simulink model "diff"  (R2023a)
settings: Solver=VariableStepAuto  StartTime=0.0  StopTime=10.0  RelTol=1e-3
libraries: slpidlib x3, embmathops x2
settings Model: Creator=Ahmed  LastModifiedBy=Ahmed

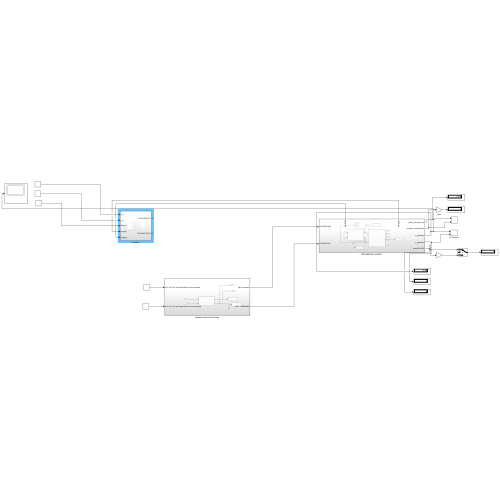
[thumbnail: Simulink's stored preview of the top-level diagram]
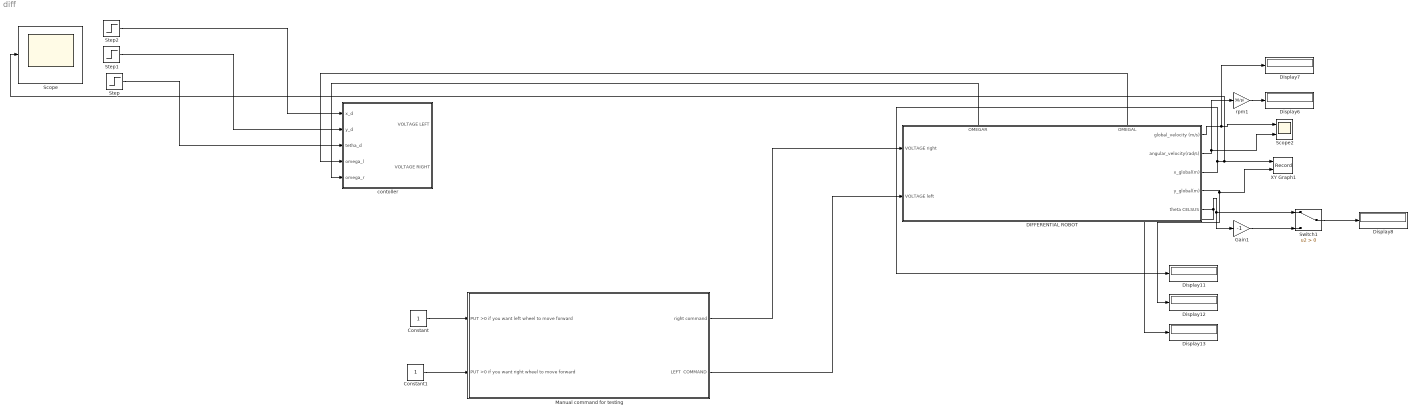
== system diff ==
  Constant : Constant
  Constant1 : Constant
  "DIFFERENTIAL ROBOT " : Subsystem
      settings: PortSchema="{\"entries\":[{\"content\":{\"sides\":[{\"content\":{\"connectorIds\":[\"In1\",\"In2\"]},\"type\":\"ConnectorPlacement.EquallySpacedRectSide\",\"uuid\":\"391234ff-cfec-4f6c-a138-89dd313d7130\"},{\"content\":{\"connectorIds\":[\"Out1\",\"Out2\",\"Out3\",\"Out4\",\"Out5\"],\"side\":\"RIGHT\"},\"type\":\"ConnectorPlacement.EquallySpacedRectSide\",\"uuid\":\"b1b937cc-f74e-4d9f-a8b8-80c8e8e7239a\"},{\"content\":{\"connectorIds\":[\"Out6\",\"Out7\"],\"side\":\"TOP\"},\"type\":\"ConnectorPlacement.EquallySpacedRectSide\",\"uuid\":\"bef0db1f-016c-4d9f-9b1d-66f8cf7cef5e\"}]},\"type\":\"ConnectorPlacement.EquallySpacedConnector\",\"uuid\":\"3118eaf9-68a7-431f-bc06-97b9db44cc22\"}],\"packageUris\":[\"http://schema.mathworks.com/mf0/Connector/R2020b\"],\"version\":\"1.0\"}"
  Display{6..8,11..13} (6 alike) : Display
  Gain1 : Gain  Gain=-1
  Manual command for testing : Subsystem
  Scope : Scope
  Scope2 : Scope  NumInputPorts=2
  Step : Step  After=0  SampleTime=0
  Step1 : Step  SampleTime=0
  Step2 : Step  SampleTime=0
  Switch1 : Switch  Criteria=u2 > Threshold  SaturateOnIntegerOverflow=off  InputSameDT=off
  XY Graph1 : Record  FileSettingsInternal="{\"entries\":[{\"content\":{\"excelSettings\":{\"content\":{},\"type\":\"Streamout.ExcelSettings\"}},\"type\":\"Streamout.FileSettingStorage\",\"uuid\":\"2b7d8dd8-c0b9-49d7-b7ba-ae24f0353f97\"}],\"packageUris\":[\"http://schema.mathworks.com/mf0/streamout_blocks/R2020a\"],\"version\":\"1.0\"}"  Layout=[1 1]  SignalsInternal="{\"entries\":[{\"content\":{\"signals\":[{\"content\":{\"blockPath\":[\"diff/XY Graph1\"],\"dimensions\":[1],\"domain\":\"diff/XY Graph1\",\"lineColor\":\"#a2142f\",\"plots\":[1],\"port\":1,\"sid\":[\"\"],\"signalID\":19857,\"signalName\":\"DIFERENTIAL ROBOT SYSTEM1:3\"},\"type\":\"RecordBlkView.Signal\",\"uuid\":\"70d8382d-8876-4a89-8d0a-8a042afd1f92\"},{\"content\":{\"blockPath\":[\"diff/XY Graph1\"],\"dimensions\":[1],\"domain\":\"diff/XY Graph1\",\"lineColor\":\"#139fff\",\"plots\":[1],\"port\":2,\"sid\":[\"\"],\"signalID\":19861,\"signalName\":\"DIFERENTIAL ROBOT SYSTEM1:4\"},\"type\":\"RecordBlkView.Signal\",\"uuid\":\"2fa1e0bd-1433-42a0-a5d9-6edbe41dc125\"}]},\"type\":\"RecordBlkView.InputSignals\",\"uuid\":\"f1bdc88a-c7a9-4fa2-8817-dae53eaa0189\"}],\"packageUris\":[\"http://schema.mathworks.com/mf0/streamout_blocks/R2020a\"],\"version\":\"1.0\"}"  VisualizationBindings="{\"xyplotplugin\":{\"info\":[{\"series\":[{\"bindingParametersList\":[{\"parameter\":\"X-Axis\",\"signalID\":19857,\"signalName\":\"DIFERENTIAL ROBOT SYSTEM1:3\"},{\"parameter\":\"Y-Axis\",\"signalID\":19861,\"signalName\":\"DIFERENTIAL ROBOT SYSTEM1:4\"}],\"seriesID\":42501}],\"subplotID\":1}]}}"  CompatibilityTag=XY
  contoller : Subsystem
  rpm1 : Gain  Gain=30/pi
  wires:
  Manual command for testing/1(right command) -> "DIFFERENTIAL ROBOT "/1(VOLTAGE right)
  Step2/1 -> contoller/1(x_d)
  Step1/1 -> contoller/2(y_d)
  Constant1/1 -> Manual command for testing/2(PUT >0 if you want right wheel to move forward)
  Step/1 -> contoller/3(tetha_d)
  "DIFFERENTIAL ROBOT "/6(OMEGAR) -> contoller/5(omega_r)
  Manual command for testing/2(LEFT  COMMAND) -> "DIFFERENTIAL ROBOT "/2(VOLTAGE left)
  "DIFFERENTIAL ROBOT "/2(angular_velocity(rad/s)) -> rpm1/1, Scope2/2
  "DIFFERENTIAL ROBOT "/1(global_velocity (m/s)) -> Display7/1, Scope2/1
  Switch1/1 -> Display8/1
  "DIFFERENTIAL ROBOT "/5(theta CELSUS) -> Gain1/1, Switch1/1, Display13/1
  Gain1/1 -> Switch1/3
  "DIFFERENTIAL ROBOT "/4(y_global(m)) -> XY Graph1/2, Display12/1
  "DIFFERENTIAL ROBOT "/7(OMEGAL) -> contoller/4(omega_l)
  rpm1/1 -> Display6/1
  "DIFFERENTIAL ROBOT "/3(x_global(m)) -> Display11/1, XY Graph1/1, Scope/1
  Constant/1 -> Manual command for testing/1(PUT >0 if you want left wheel to move forward)

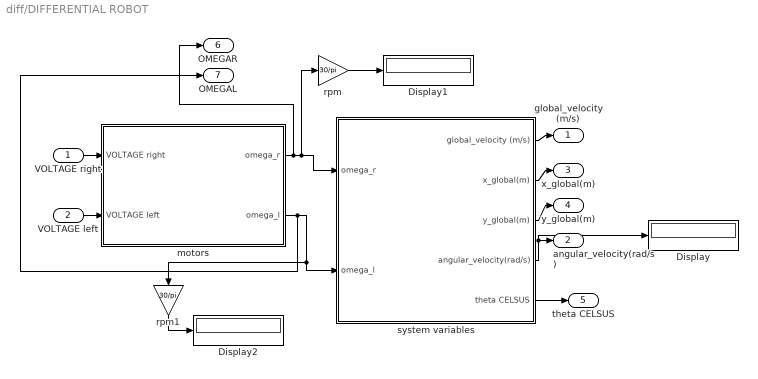
== system diff/DIFFERENTIAL ROBOT  ==
  VOLTAGE right : Inport
  VOLTAGE left : Inport  Port=2
  Display : Display
  Display1 : Display
  Display2 : Display
  motors : Subsystem
  rpm : Gain  Gain=30/pi
  rpm1 : Gain  Gain=30/pi
  system variables : Subsystem
  global_velocity (m/s) : Outport
  angular_velocity(rad/s) : Outport  Port=2
  x_global(m) : Outport  Port=3
  y_global(m) : Outport  Port=4
  theta CELSUS : Outport  Port=5
  OMEGAR : Outport  Port=6
  OMEGAL : Outport  Port=7
  wires:
  motors/1(omega_r) -> OMEGAR/1, rpm/1, system variables/1(omega_r)
  motors/2(omega_l) -> OMEGAL/1, rpm1/1, system variables/2(omega_l)
  system variables/1(global_velocity (m/s)) -> global_velocity (m/s)/1
  system variables/2(x_global(m)) -> x_global(m)/1
  system variables/3(y_global(m)) -> y_global(m)/1
  VOLTAGE right/1 -> motors/1(VOLTAGE right)
  VOLTAGE left/1 -> motors/2(VOLTAGE left)
  system variables/4(angular_velocity(rad/s)) -> Display/1, angular_velocity(rad/s)/1
  system variables/5(theta CELSUS) -> theta CELSUS/1
  rpm/1 -> Display1/1
  rpm1/1 -> Display2/1

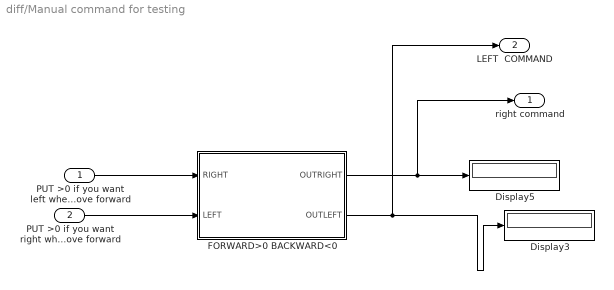
== system diff/Manual command for testing ==
  PUT >0 if you want left wheel to move forward : Inport
  PUT >0 if you want right wheel to move forward : Inport  Port=2
  Display3 : Display
  Display5 : Display
  FORWARD>0 BACKWARD<0 : Subsystem
  right command : Outport
  LEFT  COMMAND : Outport  Port=2
  wires:
  PUT >0 if you want left wheel to move forward/1 -> FORWARD>0 BACKWARD<0/1(RIGHT)
  FORWARD>0 BACKWARD<0/1(OUTRIGHT) -> right command/1, Display5/1
  FORWARD>0 BACKWARD<0/2(OUTLEFT) -> LEFT  COMMAND/1, Display3/1
  PUT >0 if you want right wheel to move forward/1 -> FORWARD>0 BACKWARD<0/2(LEFT)

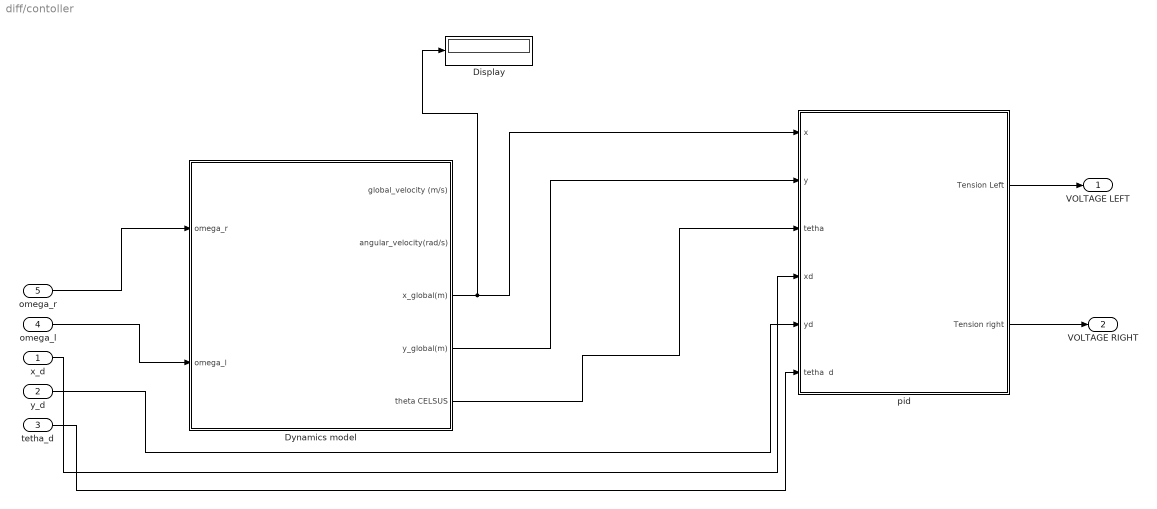
== system diff/contoller ==
  x_d : Inport
  y_d : Inport  Port=2
  tetha_d : Inport  Port=3
  omega_l : Inport  Port=4
  omega_r : Inport  Port=5
  Display : Display
  Dynamics model : Subsystem
  pid : Subsystem
  VOLTAGE LEFT : Outport
  VOLTAGE RIGHT : Outport  Port=2
  wires:
  Dynamics model/5(theta CELSUS) -> pid/3(tetha)
  Dynamics model/4(y_global(m)) -> pid/2(y)
  Dynamics model/3(x_global(m)) -> Display/1, pid/1(x)
  x_d/1 -> pid/4(xd)
  y_d/1 -> pid/5(yd)
  tetha_d/1 -> pid/6(tetha  d)
  omega_r/1 -> Dynamics model/1(omega_r)
  omega_l/1 -> Dynamics model/2(omega_l)
  pid/1(Tension Left) -> VOLTAGE LEFT/1
  pid/2(Tension right) -> VOLTAGE RIGHT/1

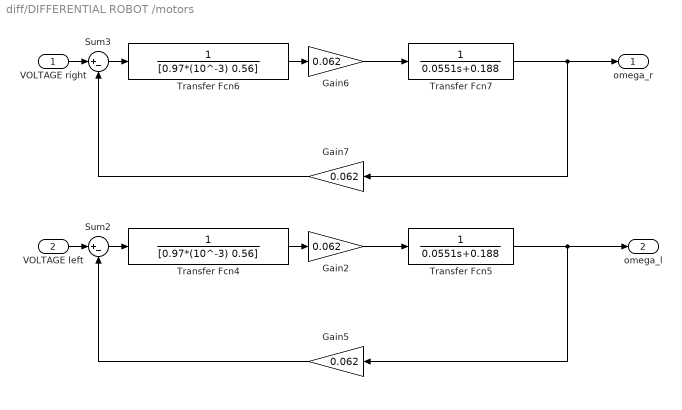
== system diff/DIFFERENTIAL ROBOT /motors ==
  VOLTAGE right : Inport
  VOLTAGE left : Inport  Port=2
  Gain{2,5..7} (4 alike) : Gain  Gain=0.062
  Sum2 : Sum  Inputs=|+-
  Sum3 : Sum  Inputs=|+-
  Transfer Fcn4 : TransferFcn  Denominator=[0.97*(10^-3) 0.56]
  Transfer Fcn5 : TransferFcn  Denominator=[0.0551 0.188]
  Transfer Fcn6 : TransferFcn  Denominator=[0.97*(10^-3) 0.56]
  Transfer Fcn7 : TransferFcn  Denominator=[0.0551 0.188]
  omega_r : Outport
  omega_l : Outport  Port=2
  wires:
  Transfer Fcn7/1 -> omega_r/1, Gain7/1
  Gain2/1 -> Transfer Fcn5/1
  Transfer Fcn5/1 -> omega_l/1, Gain5/1
  Gain6/1 -> Transfer Fcn7/1
  VOLTAGE left/1 -> Sum2/1
  Sum2/1 -> Transfer Fcn4/1
  Transfer Fcn6/1 -> Gain6/1
  Sum3/1 -> Transfer Fcn6/1
  Gain5/1 -> Sum2/2
  VOLTAGE right/1 -> Sum3/1
  Gain7/1 -> Sum3/2
  Transfer Fcn4/1 -> Gain2/1

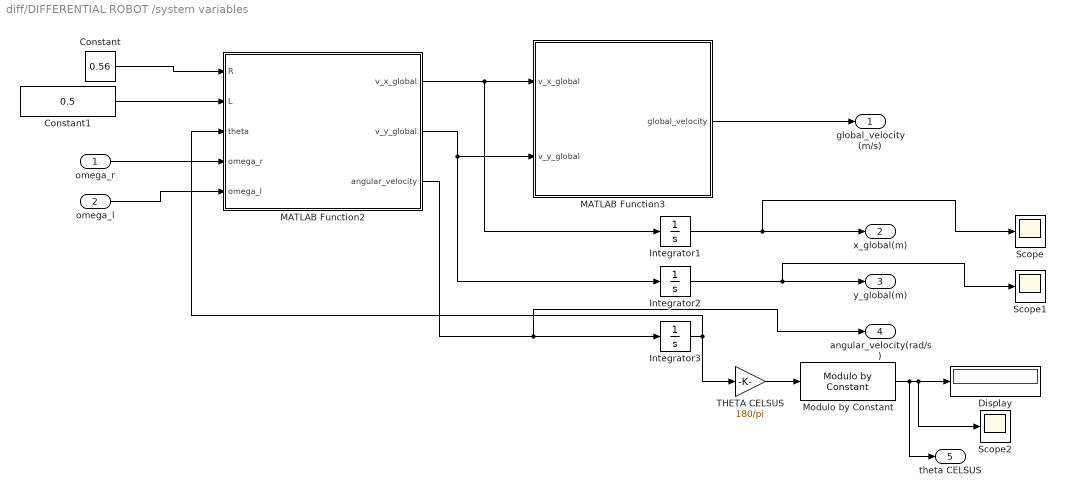
== system diff/DIFFERENTIAL ROBOT /system variables ==
  omega_r : Inport
  omega_l : Inport  Port=2
  Constant : Constant  Value=0.56
  Constant1 : Constant  Value=0.5
  Display : Display
  Integrator1 : Integrator
  Integrator2 : Integrator
  Integrator3 : Integrator
  MATLAB Function2 : MATLAB Function  TreatAsAtomicUnit=on
  MATLAB Function3 : MATLAB Function  TreatAsAtomicUnit=on
  Modulo by Constant : embmathops/Modulo by Constant  Denominator=360  SimulateUsing=Code generation
      settings: LibrarySourceBlock=embeddedMathLib/Modulo by Constant
  Scope : Scope
  Scope1 : Scope
  Scope2 : Scope
  THETA CELSUS : Gain  Gain=180/pi
  global_velocity (m/s) : Outport
  x_global(m) : Outport  Port=2
  y_global(m) : Outport  Port=3
  angular_velocity(rad/s) : Outport  Port=4
  theta CELSUS : Outport  Port=5
  wires:
  MATLAB Function2/3(angular_velocity) -> angular_velocity(rad/s)/1, Integrator3/1
  MATLAB Function2/1(v_x_global) -> Integrator1/1, MATLAB Function3/1(v_x_global)
  Constant1/1 -> MATLAB Function2/2(L)
  Integrator3/1 -> MATLAB Function2/3(theta), THETA CELSUS/1
  omega_l/1 -> MATLAB Function2/5(omega_l)
  MATLAB Function2/2(v_y_global) -> Integrator2/1, MATLAB Function3/2(v_y_global)
  Constant/1 -> MATLAB Function2/1(R)
  omega_r/1 -> MATLAB Function2/4(omega_r)
  Integrator2/1 -> Scope1/1, y_global(m)/1
  Integrator1/1 -> Scope/1, x_global(m)/1
  MATLAB Function3/1(global_velocity) -> global_velocity (m/s)/1
  Modulo by Constant/1 -> theta CELSUS/1, Display/1, Scope2/1
  THETA CELSUS/1 -> Modulo by Constant/1

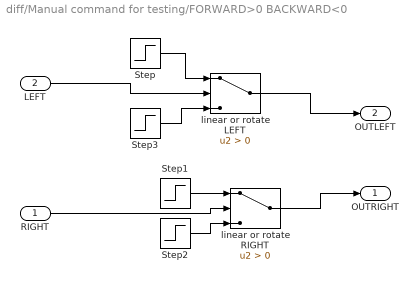
== system diff/Manual command for testing/FORWARD>0 BACKWARD<0 ==
  RIGHT : Inport
  LEFT : Inport  Port=2
  Step : Step  After=12  SampleTime=0
  Step1 : Step  After=12  SampleTime=0
  Step2 : Step  After=-12  SampleTime=0
  Step3 : Step  After=-12  SampleTime=0
  linear or rotate LEFT : Switch  Criteria=u2 > Threshold  SaturateOnIntegerOverflow=off  InputSameDT=off
  "linear or rotate RIGHT " : Switch  Criteria=u2 > Threshold  SaturateOnIntegerOverflow=off  InputSameDT=off
  OUTRIGHT : Outport
  OUTLEFT : Outport  Port=2
  wires:
  Step1/1 -> "linear or rotate RIGHT "/1
  "linear or rotate RIGHT "/1 -> OUTRIGHT/1
  Step2/1 -> "linear or rotate RIGHT "/3
  RIGHT/1 -> "linear or rotate RIGHT "/2
  Step3/1 -> linear or rotate LEFT/3
  Step/1 -> linear or rotate LEFT/1
  linear or rotate LEFT/1 -> OUTLEFT/1
  LEFT/1 -> linear or rotate LEFT/2

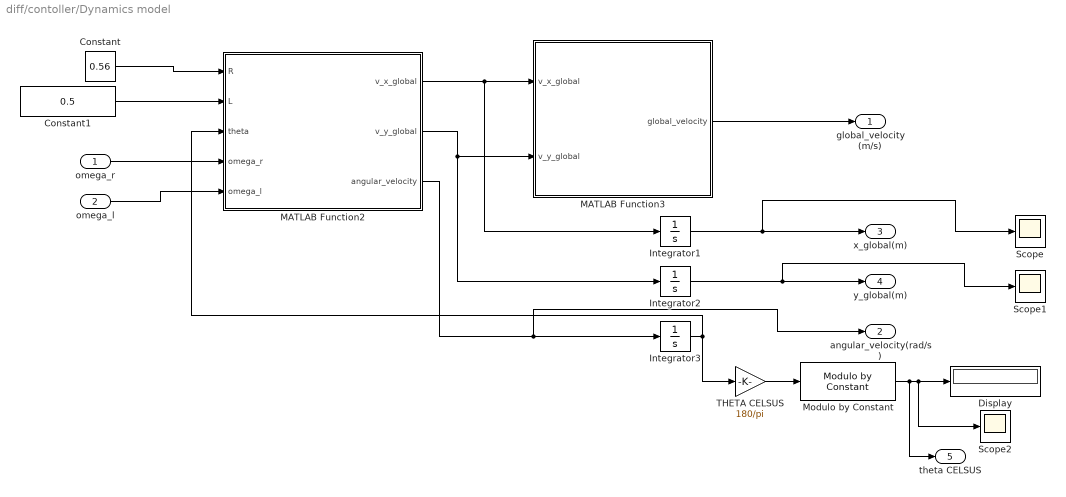
== system diff/contoller/Dynamics model ==
  omega_r : Inport
  omega_l : Inport  Port=2
  Constant : Constant  Value=0.56
  Constant1 : Constant  Value=0.5
  Display : Display
  Integrator1 : Integrator
  Integrator2 : Integrator
  Integrator3 : Integrator
  MATLAB Function2 : MATLAB Function  TreatAsAtomicUnit=on
  MATLAB Function3 : MATLAB Function  TreatAsAtomicUnit=on
  Modulo by Constant : embmathops/Modulo by Constant  Denominator=360  SimulateUsing=Code generation
      settings: LibrarySourceBlock=embeddedMathLib/Modulo by Constant
  Scope : Scope
  Scope1 : Scope
  Scope2 : Scope
  THETA CELSUS : Gain  Gain=180/pi
  global_velocity (m/s) : Outport
  angular_velocity(rad/s) : Outport  Port=2
  x_global(m) : Outport  Port=3
  y_global(m) : Outport  Port=4
  theta CELSUS : Outport  Port=5
  wires:
  MATLAB Function2/3(angular_velocity) -> angular_velocity(rad/s)/1, Integrator3/1
  MATLAB Function2/1(v_x_global) -> Integrator1/1, MATLAB Function3/1(v_x_global)
  Constant1/1 -> MATLAB Function2/2(L)
  Integrator3/1 -> MATLAB Function2/3(theta), THETA CELSUS/1
  omega_l/1 -> MATLAB Function2/5(omega_l)
  MATLAB Function2/2(v_y_global) -> Integrator2/1, MATLAB Function3/2(v_y_global)
  Constant/1 -> MATLAB Function2/1(R)
  omega_r/1 -> MATLAB Function2/4(omega_r)
  Integrator2/1 -> Scope1/1, y_global(m)/1
  Integrator1/1 -> Scope/1, x_global(m)/1
  MATLAB Function3/1(global_velocity) -> global_velocity (m/s)/1
  Modulo by Constant/1 -> theta CELSUS/1, Display/1, Scope2/1
  THETA CELSUS/1 -> Modulo by Constant/1

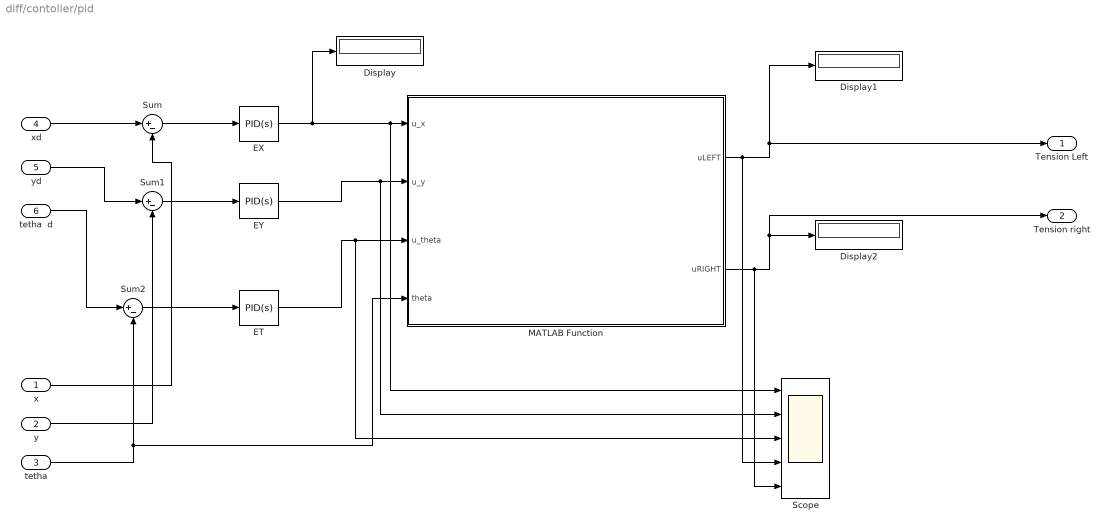
== system diff/contoller/pid ==
  x : Inport
  y : Inport  Port=2
  tetha : Inport  Port=3
  xd : Inport  Port=4
  yd : Inport  Port=5
  tetha  d : Inport  Port=6
  Display : Display
  Display1 : Display
  Display2 : Display
  ET : slpidlib/PID Controller  Controller=PID  Form=Parallel  TimeDomain=Continuous-time  UseExternalTs=off  SampleTime=-1  IntegratorMethod=Forward Euler  FilterMethod=Forward Euler  ControllerParametersSource=internal  P=1  I=0  UseKiTs=off  D=0  N=100  UseFilter=on  TunerSelectOption=Transfer Function Based (PID Tuner App)  InitialConditionSource=internal  InitialConditionForIntegrator=0  InitialConditionForFilter=0  DifferentiatorICPrevScaledInput=0  ExternalReset=none  TrackingMode=off  Kt=1  LimitOutput=off  SatLimitsSource=internal  UpperSaturationLimit=inf  LowerSaturationLimit=-inf  LinearizeAsGain=on  AntiWindupMode=none  Kb=1  LimitIntegrator=off  UpperIntegratorSaturationLimit=inf  LowerIntegratorSaturationLimit=-inf  POutMin=[]  POutMax=[]  IOutMin=[]  IOutMax=[]  DOutMin=[]  DOutMax=[]  NOutMin=[]  NOutMax=[]  SumOutMin=[]  SumOutMax=[]  SaturationOutMin=[]  SaturationOutMax=[]  PParamMin=[]  PParamMax=[]  IParamMin=[]  IParamMax=[]  DParamMin=[]  DParamMax=[]  NParamMin=[]  NParamMax=[]  KbParamMin=[]  KbParamMax=[]  KtParamMin=[]  KtParamMax=[]  KbOutMin=[]  KbOutMax=[]  KtOutMin=[]  KtOutMax=[]  IntegratorOutMin=[]  IntegratorOutMax=[]  FilterOutMin=[]  FilterOutMax=[]  SumI1OutMin=[]  SumI1OutMax=[]  SumI2OutMin=[]  SumI2OutMax=[]  SumI3OutMin=[]  SumI3OutMax=[]  SumI4OutMin=[]  SumI4OutMax=[]  SumDOutMin=[]  SumDOutMax=[]  DifferentiatorOutMin=[]  DifferentiatorOutMax=[]  FilterDiffOutCoefMin=[]  FilterDiffOutCoefMax=[]  ReciprocalOutMin=[]  ReciprocalOutMax=[]  SumDenOutMin=[]  SumDenOutMax=[]  SumNumOutMin=[]  SumNumOutMax=[]  DivideOutMin=[]  DivideOutMax=[]  UdiffTsProdOutMin=[]  UdiffTsProdOutMax=[]  NTsProdOutMin=[]  NTsProdOutMax=[]  UintegralTsProdOutMin=[]  UintegralTsProdOutMax=[]  UngainTsProdOutMin=[]  UngainTsProdOutMax=[]  ClampingZeroOutDataTypeStr=Inherit: Inherit via back propagation  ClampingZeroOutMin=[]  ClampingZeroOutMax=[]  FilterDenConstantOutDataTypeStr=Inherit: Inherit via back propagation  FilterDenConstantOutMin=[]  FilterDenConstantOutMax=[]  PCopyOutDataTypeStr=Inherit: Inherit via back propagation  PCopyOutMin=[]  PCopyOutMax=[]  NCopyOutDataTypeStr=Inherit: Inherit via back propagation  NCopyOutMin=[]  NCopyOutMax=[]  IntegratorContinuousStateAttributes=''  IntegratorStateMustResolveToSignalObject=off  IntegratorRTWStateStorageClass=Auto  FilterContinuousStateAttributes=''  FilterStateMustResolveToSignalObject=off  FilterRTWStateStorageClass=Auto  ParallelPVariant=InternalParameters  IdealPVariant=Disabled  IVariant=InternalParameters  DVariant=InternalParameters  IntegratorVariant=Continuous  SatVariant=Disabled  AWVariant=Passthrough  PCopyVariant=Disabled  TRVariant=Disabled  FdbkBlocksVariant=Forward  IdealPFdbkVariant=Disabled  SatFdbkVariant=Disabled  DerivativeFilterVariant=ContFilter  NVariant=InternalParameters  NCopyVariant=Disabled  FilterICVariant=InternalICsFilter  IntegratorICVariant=InternalICs  ExternalResetVariant=Disabled  TRSumVariant=Passthrough  SumFdbkVariant=Disabled  SumVariant=Sum_PID  TsampFilterVariant=InternalTs  TsampNgainVariant=Passthrough  TsampIntegralVariant=Disabled_SignalSpec  ExternalSaturationOutDataTypeStr=Inherit: Same as second input
  EX : slpidlib/PID Controller  Controller=PID  Form=Parallel  TimeDomain=Continuous-time  UseExternalTs=off  SampleTime=-1  IntegratorMethod=Forward Euler  FilterMethod=Forward Euler  ControllerParametersSource=internal  P=3.6  I=5  UseKiTs=off  D=0.5  N=100  UseFilter=on  TunerSelectOption=Transfer Function Based (PID Tuner App)  InitialConditionSource=internal  InitialConditionForIntegrator=0  InitialConditionForFilter=0  DifferentiatorICPrevScaledInput=0  ExternalReset=none  TrackingMode=off  Kt=1  LimitOutput=off  SatLimitsSource=internal  UpperSaturationLimit=inf  LowerSaturationLimit=-inf  LinearizeAsGain=on  AntiWindupMode=none  Kb=1  LimitIntegrator=off  UpperIntegratorSaturationLimit=inf  LowerIntegratorSaturationLimit=-inf  POutMin=[]  POutMax=[]  IOutMin=[]  IOutMax=[]  DOutMin=[]  DOutMax=[]  NOutMin=[]  NOutMax=[]  SumOutMin=[]  SumOutMax=[]  SaturationOutMin=[]  SaturationOutMax=[]  PParamMin=[]  PParamMax=[]  IParamMin=[]  IParamMax=[]  DParamMin=[]  DParamMax=[]  NParamMin=[]  NParamMax=[]  KbParamMin=[]  KbParamMax=[]  KtParamMin=[]  KtParamMax=[]  KbOutMin=[]  KbOutMax=[]  KtOutMin=[]  KtOutMax=[]  IntegratorOutMin=[]  IntegratorOutMax=[]  FilterOutMin=[]  FilterOutMax=[]  SumI1OutMin=[]  SumI1OutMax=[]  SumI2OutMin=[]  SumI2OutMax=[]  SumI3OutMin=[]  SumI3OutMax=[]  SumI4OutMin=[]  SumI4OutMax=[]  SumDOutMin=[]  SumDOutMax=[]  DifferentiatorOutMin=[]  DifferentiatorOutMax=[]  FilterDiffOutCoefMin=[]  FilterDiffOutCoefMax=[]  ReciprocalOutMin=[]  ReciprocalOutMax=[]  SumDenOutMin=[]  SumDenOutMax=[]  SumNumOutMin=[]  SumNumOutMax=[]  DivideOutMin=[]  DivideOutMax=[]  UdiffTsProdOutMin=[]  UdiffTsProdOutMax=[]  NTsProdOutMin=[]  NTsProdOutMax=[]  UintegralTsProdOutMin=[]  UintegralTsProdOutMax=[]  UngainTsProdOutMin=[]  UngainTsProdOutMax=[]  ClampingZeroOutDataTypeStr=Inherit: Inherit via back propagation  ClampingZeroOutMin=[]  ClampingZeroOutMax=[]  FilterDenConstantOutDataTypeStr=Inherit: Inherit via back propagation  FilterDenConstantOutMin=[]  FilterDenConstantOutMax=[]  PCopyOutDataTypeStr=Inherit: Inherit via back propagation  PCopyOutMin=[]  PCopyOutMax=[]  NCopyOutDataTypeStr=Inherit: Inherit via back propagation  NCopyOutMin=[]  NCopyOutMax=[]  IntegratorContinuousStateAttributes=''  IntegratorStateMustResolveToSignalObject=off  IntegratorRTWStateStorageClass=Auto  FilterContinuousStateAttributes=''  FilterStateMustResolveToSignalObject=off  FilterRTWStateStorageClass=Auto  ParallelPVariant=InternalParameters  IdealPVariant=Disabled  IVariant=InternalParameters  DVariant=InternalParameters  IntegratorVariant=Continuous  SatVariant=Disabled  AWVariant=Passthrough  PCopyVariant=Disabled  TRVariant=Disabled  FdbkBlocksVariant=Forward  IdealPFdbkVariant=Disabled  SatFdbkVariant=Disabled  DerivativeFilterVariant=ContFilter  NVariant=InternalParameters  NCopyVariant=Disabled  FilterICVariant=InternalICsFilter  IntegratorICVariant=InternalICs  ExternalResetVariant=Disabled  TRSumVariant=Passthrough  SumFdbkVariant=Disabled  SumVariant=Sum_PID  TsampFilterVariant=InternalTs  TsampNgainVariant=Passthrough  TsampIntegralVariant=Disabled_SignalSpec  ExternalSaturationOutDataTypeStr=Inherit: Same as second input
  EY : slpidlib/PID Controller  Controller=PID  Form=Parallel  TimeDomain=Continuous-time  UseExternalTs=off  SampleTime=-1  IntegratorMethod=Forward Euler  FilterMethod=Forward Euler  ControllerParametersSource=internal  P=1  I=0  UseKiTs=off  D=0  N=100  UseFilter=on  TunerSelectOption=Transfer Function Based (PID Tuner App)  InitialConditionSource=internal  InitialConditionForIntegrator=0  InitialConditionForFilter=0  DifferentiatorICPrevScaledInput=0  ExternalReset=none  TrackingMode=off  Kt=1  LimitOutput=off  SatLimitsSource=internal  UpperSaturationLimit=inf  LowerSaturationLimit=-inf  LinearizeAsGain=on  AntiWindupMode=none  Kb=1  LimitIntegrator=off  UpperIntegratorSaturationLimit=inf  LowerIntegratorSaturationLimit=-inf  POutMin=[]  POutMax=[]  IOutMin=[]  IOutMax=[]  DOutMin=[]  DOutMax=[]  NOutMin=[]  NOutMax=[]  SumOutMin=[]  SumOutMax=[]  SaturationOutMin=[]  SaturationOutMax=[]  PParamMin=[]  PParamMax=[]  IParamMin=[]  IParamMax=[]  DParamMin=[]  DParamMax=[]  NParamMin=[]  NParamMax=[]  KbParamMin=[]  KbParamMax=[]  KtParamMin=[]  KtParamMax=[]  KbOutMin=[]  KbOutMax=[]  KtOutMin=[]  KtOutMax=[]  IntegratorOutMin=[]  IntegratorOutMax=[]  FilterOutMin=[]  FilterOutMax=[]  SumI1OutMin=[]  SumI1OutMax=[]  SumI2OutMin=[]  SumI2OutMax=[]  SumI3OutMin=[]  SumI3OutMax=[]  SumI4OutMin=[]  SumI4OutMax=[]  SumDOutMin=[]  SumDOutMax=[]  DifferentiatorOutMin=[]  DifferentiatorOutMax=[]  FilterDiffOutCoefMin=[]  FilterDiffOutCoefMax=[]  ReciprocalOutMin=[]  ReciprocalOutMax=[]  SumDenOutMin=[]  SumDenOutMax=[]  SumNumOutMin=[]  SumNumOutMax=[]  DivideOutMin=[]  DivideOutMax=[]  UdiffTsProdOutMin=[]  UdiffTsProdOutMax=[]  NTsProdOutMin=[]  NTsProdOutMax=[]  UintegralTsProdOutMin=[]  UintegralTsProdOutMax=[]  UngainTsProdOutMin=[]  UngainTsProdOutMax=[]  ClampingZeroOutDataTypeStr=Inherit: Inherit via back propagation  ClampingZeroOutMin=[]  ClampingZeroOutMax=[]  FilterDenConstantOutDataTypeStr=Inherit: Inherit via back propagation  FilterDenConstantOutMin=[]  FilterDenConstantOutMax=[]  PCopyOutDataTypeStr=Inherit: Inherit via back propagation  PCopyOutMin=[]  PCopyOutMax=[]  NCopyOutDataTypeStr=Inherit: Inherit via back propagation  NCopyOutMin=[]  NCopyOutMax=[]  IntegratorContinuousStateAttributes=''  IntegratorStateMustResolveToSignalObject=off  IntegratorRTWStateStorageClass=Auto  FilterContinuousStateAttributes=''  FilterStateMustResolveToSignalObject=off  FilterRTWStateStorageClass=Auto  ParallelPVariant=InternalParameters  IdealPVariant=Disabled  IVariant=InternalParameters  DVariant=InternalParameters  IntegratorVariant=Continuous  SatVariant=Disabled  AWVariant=Passthrough  PCopyVariant=Disabled  TRVariant=Disabled  FdbkBlocksVariant=Forward  IdealPFdbkVariant=Disabled  SatFdbkVariant=Disabled  DerivativeFilterVariant=ContFilter  NVariant=InternalParameters  NCopyVariant=Disabled  FilterICVariant=InternalICsFilter  IntegratorICVariant=InternalICs  ExternalResetVariant=Disabled  TRSumVariant=Passthrough  SumFdbkVariant=Disabled  SumVariant=Sum_PID  TsampFilterVariant=InternalTs  TsampNgainVariant=Passthrough  TsampIntegralVariant=Disabled_SignalSpec  ExternalSaturationOutDataTypeStr=Inherit: Same as second input
  MATLAB Function : MATLAB Function  TreatAsAtomicUnit=on
  Scope : Scope  NumInputPorts=5
  Sum : Sum  Inputs=|+-
  Sum1 : Sum  Inputs=|+-
  Sum2 : Sum  Inputs=|+-
  Tension Left : Outport
  Tension right : Outport  Port=2
  wires:
  xd/1 -> Sum/1
  yd/1 -> Sum1/1
  tetha  d/1 -> Sum2/1
  x/1 -> Sum/2
  y/1 -> Sum1/2
  tetha/1 -> MATLAB Function/4(theta), Sum2/2
  Sum1/1 -> EY/1
  Sum/1 -> EX/1
  Sum2/1 -> ET/1
  EX/1 -> Display/1, Scope/1, MATLAB Function/1(u_x)
  EY/1 -> Scope/2, MATLAB Function/2(u_y)
  ET/1 -> Scope/3, MATLAB Function/3(u_theta)
  MATLAB Function/1(uLEFT) -> Scope/4, Tension Left/1, Display1/1
  MATLAB Function/2(uRIGHT) -> Scope/5, Tension right/1, Display2/1

== matlab function diff/DIFFERENTIAL ROBOT /system variables/MATLAB Function2 ==
  data: v_x_global output; v_y_global output; R input; L input; theta input; omega_r input; omega_l input; angular_velocity output
function [v_x_global, v_y_global, angular_velocity] = robotKinematics(R, L, theta, omega_r, omega_l)
    % Inputs:
    % R: Radius of the wheels (meters)
    % L: Distance between the wheels (meters)
    % theta: Current orientation of the robot (in radians)
    % omega_r: Angular velocity of the right wheel (rad/s)
    % omega_l: Angular velocity of the left wheel (rad/s)
    
    % Transformation matrix
    T = [R/2 * cos(theta), R/2 * cos(theta);
         R/2 * sin(theta), R/2 * sin(theta);
         R/L,            -R/L];
     
    % Wheel angular velocity vector
    omega = [omega_r; omega_l];
    
    % Compute velocity components
    q_i = T * omega;
    
    % Extract components
    v_x_global = q_i(1);          % Global linear velocity in x-direction
    v_y_global = q_i(2);          % Global linear velocity in y-direction
    angular_velocity = q_i(3);  % Angular velocity (theta_dot)
end

== matlab function diff/DIFFERENTIAL ROBOT /system variables/MATLAB Function3 ==
  data: v_x_global input; global_velocity output; v_y_global input
function global_velocity  = calculateGlobalVelocity(v_x_global, v_y_global)
    % Inputs:
    % x_global: Global linear velocity in x-direction (m/s)
    % y_global: Global linear velocity in y-direction (m/s)
    
    % Compute the magnitude of the global velocity
    global_velocity = sqrt(v_x_global^2 + v_y_global^2);
    
   
end

== matlab function diff/contoller/Dynamics model/MATLAB Function2 ==
  data: v_x_global output; v_y_global output; R input; L input; theta input; omega_r input; omega_l input; angular_velocity output
function [v_x_global, v_y_global, angular_velocity] = robotKinematics(R, L, theta, omega_r, omega_l)
    % Inputs:
    % R: Radius of the wheels (meters)
    % L: Distance between the wheels (meters)
    % theta: Current orientation of the robot (in radians)
    % omega_r: Angular velocity of the right wheel (rad/s)
    % omega_l: Angular velocity of the left wheel (rad/s)
    
    % Transformation matrix
    T = [R/2 * cos(theta), R/2 * cos(theta);
         R/2 * sin(theta), R/2 * sin(theta);
         R/L,            -R/L];
     
    % Wheel angular velocity vector
    omega = [omega_r; omega_l];
    
    % Compute velocity components
    q_i = T * omega;
    
    % Extract components
    v_x_global = q_i(1);          % Global linear velocity in x-direction
    v_y_global = q_i(2);          % Global linear velocity in y-direction
    angular_velocity = q_i(3);  % Angular velocity (theta_dot)
end

== matlab function diff/contoller/Dynamics model/MATLAB Function3 ==
  data: v_x_global input; global_velocity output; v_y_global input
function global_velocity  = calculateGlobalVelocity(v_x_global, v_y_global)
    % Inputs:
    % x_global: Global linear velocity in x-direction (m/s)
    % y_global: Global linear velocity in y-direction (m/s)
    
    % Compute the magnitude of the global velocity
    global_velocity = sqrt(v_x_global^2 + v_y_global^2);
    
   
end

== matlab function diff/contoller/pid/MATLAB Function ==
  data: u_x input; uLEFT output; u_y input; u_theta input; theta input; uRIGHT output
function [uLEFT, uRIGHT] = MIMO_PID_control(u_x, u_y, u_theta, theta)
    % MIMO PID Control for a differential drive robot
    % Inputs:
    % u_x      - Desired linear velocity in the x direction
    % u_y      - Desired linear velocity in the y direction
    % u_theta  - Desired angular velocity (theta)
    % r        - Wheel radius
    % L        - Distance between wheels (wheelbase)
    % theta    - Current robot orientation (theta)
    R=0.5;
    L=0.127;
    % Compute the motor velocities based on kinematics
    % Using the derived equations:
    % u1 = (1/2) * ( (2/r) * (u_x * cos(theta) + u_y * sin(theta)) + (L/r) * u_theta )
    % u2 = (1/2) * ( (2/r) * (u_x * cos(theta) + u_y * sin(theta)) - (L/r) * u_theta )
    
    % Term for the linear velocities in the x and y directions
    linear_term = (2 / R ) * (u_x * cos(theta) + u_y * sin(theta));
    
    % Compute the left and right motor velocities
    uLEFT = 0.5 * (linear_term + (L / R ) * u_theta);
    uRIGHT = 0.5 * (linear_term - (L / R ) * u_theta);
    
    % Return the calculated motor inputs
end
